simulink model "sdl_gear_efficiency"  (R2019b)
settings: Solver=VariableStepAuto  StartTime=0.0  StopTime=10  FixedStep=0.01  RelTol=1e-3  AbsTol=1e-3  EnableMultiTasking=on
undefined symbols (not defined in the file): sigbuilder_block
libraries: fl_lib x6, nesl_utility x5, sdl_lib x3
CloseFcn:
  | try,close(h1_sdl_gear_efficiency),end
  | clear h1_sdl_gear_efficiency
  | 
  | 
  | clear simlog_sdl_gear_efficiency
  | clear logsout_sdl_gear_efficiency
Description:
  | Gearbox Efficiency Measurement
settings Model: Creator=MathWorks  LastModifiedBy=JPark
settings SolverCC: AutoScaleAbsTol=off  MaxConsecutiveMinStep=5
settings DataIOCC: LimitDataPoints=on  MaxDataPoints=10000  SaveOutput=off  DSMLogging=off  SaveTime=off  ReturnWorkspaceOutputs=off  SignalLoggingName=logsout_sdl_gear_efficiency
settings OptimizationCC: ExpressionDepthLimit=2147483647  EfficientMapNaN2IntZero=off  LifeSpan=inf
settings DebuggingCC: StateNameClashWarn=warning  PregeneratedLibrarySubsystemCodeDiagnostic=none  SFUnexpectedBacktrackingDiag=warning  SFNoUnconditionalDefaultTransitionDiag=warning  SFExecutionAtInitializationDiag=none  ArithmeticOperatorsInVariantConditions=warning
settings HardwareCC: ProdBitPerPointer=32  ProdBitPerSizeT=32  ProdBitPerPtrDiffT=32  ProdLargestAtomicFloat=None  ProdIntDivRoundTo=Undefined  ProdEndianess=Unspecified  ProdWordSize=32  ProdHWDeviceType=32-bit Generic
settings ModelReferenceCC: PropagateSignalLabelsOutOfModel=off
settings SFSimCC: SimUseLocalCustomCode=off  CustomCodeUndefinedFunction=UseInterfaceOnly
settings RTWCC: RTWUseLocalCustomCode=off
settings CodeAppCC: StateflowObjectComments=on
settings GRTTargetCC: TargetLangStandard=C89/C90 (ANSI)  GeneratePreprocessorConditionals=Disable all  CombineOutputUpdateFcns=off  GRTInterface=on
settings ConfigComp: CovMetricSettings=dw  CovHtmlReporting=on  CovSaveCumulativeToWorkspaceVar=on  CovSaveSingleToWorkspaceVar=on  CovShowResultsExplorer=off  CovExternalEMLEnable=off
settings SimscapeCC: SimscapeLogType=all  SimscapeLogSimulationStatistics=on  SimscapeLogName=simlog_sdl_gear_efficiency  SimscapeLogDataHistory=10000

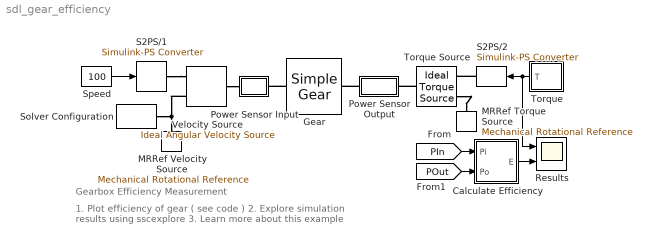
== system sdl_gear_efficiency ==
  note: Gearbox Efficiency Measurement
  note: 1. Plot efficiency of gear ( see code )
      | 2. Explore simulation results using sscexplore
      | 3. Learn more about this example
  Calculate Efficiency : Subsystem
  Gear : sdl_lib/Gears/Simple Gear  ratio=6.3  rotation_direction=1  friction_model=3  T_noload=2.4 N*m  T_nom=150 N*m  efficiency_nom=0.8  efficiency=0.8  mu_visc=[ 1e-5 1e-5 ] N*m/(rad/s)  w_thr=0.01 rad/s  pwr_thr=0.001 W  enable_faults=simscape.enum.onoff.off  efficiency_fault=0.05  external_fault=simscape.enum.onoff.off  temporal_fault=simscape.enum.onoff.off  fault_time=5 s  fault_angles=pi / 12 rad  report_fault=1  temperature_TLU=[ 280 300 320 ] K  load_TLU=[ 1 5 10 ] N*m  efficiency_TLU=[ 0.95 0.9 0.85 ]  efficiency_TLU2=[ 0.85 0.8 0.75; 0.95 0.9 0.85; 0.85 0.8 0.7 ]  thermal_mass=50 J/K  T_init=300 K
      settings: SourceProductName=Simscape Driveline
      settings: AttributesFormatString=|
      | Nominal Efficiency: %<efficiency_nom>
      | Nominal Output Torque: %<T_nom> %<T_nom_unit>
  MRRef Torque Source : fl_lib/Mechanical/Rotational Elements/Mechanical Rotational Reference
  MRRef Velocity Source : fl_lib/Mechanical/Rotational Elements/Mechanical Rotational Reference
  Power Sensor Input : Subsystem
      mask Display: disp('PIn');
  Power Sensor Output : Subsystem
      mask Display: disp('POut');
  Results : Scope  NumInputPorts=2
  S2PS/1 : nesl_utility/Simulink-PS Converter  PhysicalDomain=network_engine_domain  SubClassName=ps_input  LeftPortType=input  RightPortType=output  PseudoPeriodic=off  Frequencies=[]  NoiseDistribution=none  NoiseParameters=[]  Unit=rad/s  AffineConversion=off  FilteringAndDerivatives=zero  SimscapeFilterOrder=1  InputFilterTimeConstant=.001  UdotUserProvided=0
  S2PS/2 : nesl_utility/Simulink-PS Converter  PhysicalDomain=network_engine_domain  SubClassName=ps_input  LeftPortType=input  RightPortType=output  PseudoPeriodic=off  Frequencies=[]  NoiseDistribution=none  NoiseParameters=[]  Unit=N*m  AffineConversion=off  FilteringAndDerivatives=zero  SimscapeFilterOrder=1  InputFilterTimeConstant=.001  UdotUserProvided=0
  Solver Configuration : nesl_utility/Solver Configuration  PhysicalDomain=network_engine_domain  SubClassName=solver  LeftPortType=input  RightPortType=generic  Tones=[]  Harmonics=[]  SimulateNoise=off  Profile=off  UseLocalSampling=off  EnableSwitchedLinearOptims=on  FrequencyDomain=off  UseCCode=off  RelTol=0.001  AbsTol=1e-06  MinStep=1e-09  ToWorkspace=off  RevertToSquareIcSolve=off  NumHomotopyIterations=100  PhasorMode=off  PhasorModeNumHarmonics=1  DoDC=off  ResidualTolerance=1e-9  UseLocalSolver=off  LocalSolverChoice=NE_PARTITIONING_ADVANCER  LocalSolverSampleTime=0.01  DoFixedCost=off  MaxNonlinIter=3  MaxModeIter=2  LinearAlgebra=auto  EquationFormulation=NE_TIME_EF  DelaysMemoryBudget=1024  AutomaticFiltering=on  FilteringTimeConstant=0.001  PartitionStorageMethod=EXHAUSTIVE  PartitionMemoryBudget=1024  PartitionMethod=ROBUST
  Speed : Constant  Value=100
  Torque : Subsystem  Tag=STV Subsys  LoadFcn=sigbuilder_block('load');  StartFcn=sigbuilder_block('start');  StopFcn=sigbuilder_block('stop');  ClipboardFcn=sigbuilder_block('clipboard');  mask(Sigbuilder block){tuvar=[0:10]}
      mask help: Sigbuilder GUI
      mask init:
      | if ~strcmp(get_param(bdroot(gcbh),'SimulationStatus'),'stopped') tuvar = sigbuilder_block('maskInit'); end
      settings: CopyFcn=sigbuilder_block('copy');  DeleteFcn=sigbuilder_block('delete');  ModelCloseFcn=sigbuilder_block('modelClose');  PreSaveFcn=sigbuilder_block('preSave');  PauseFcn=sigbuilder_block('pause')  ContinueFcn=sigbuilder_block('continue')  NameChangeFcn=sigbuilder_block('namechange');  OpenFcn=sigbuilder_block('open',[301.2 157.5 550.2 398.4 ]);  CloseFcn=sigbuilder_block('close');
      mask Display: plot(0, 0, 100, 100,[2, 2, 32, 32, 2], [68, 8, 8, 68, 68],[32, 2], [38, 38], [32, 19, 2],[53, 60, 44], [32, 17, 17, 2],[16, 16, 31, 31]);txt = getActiveGroup(gcbh);text(2, 100, txt,'verticalAlignment', 'top');
  Torque Source : fl_lib/Mechanical/Mechanical Sources/Ideal Torque Source
  Velocity Source : fl_lib/Mechanical/Mechanical Sources/Ideal Angular Velocity Source
  wires:
  Speed/1 -> S2PS/1/1
  [PIn] -> Calculate Efficiency/1(Pi)
  Torque/1(T) -> Results/1, S2PS/2/1
  [POut] -> Calculate Efficiency/2(Po)
  Calculate Efficiency/1(E) -> Results/2
  connections:
  Velocity Source/LConn1 -- Power Sensor Input/LConn1
  S2PS/1/RConn1 -- Velocity Source/RConn1
  Velocity Source/RConn2 -- Solver Configuration/RConn1 -- MRRef Velocity Source/LConn1
  Torque Source/RConn2 -- MRRef Torque Source/LConn1
  Gear/LConn1 -- Power Sensor Input/RConn1
  Power Sensor Output/LConn1 -- Gear/RConn1
  S2PS/2/RConn1 -- Torque Source/RConn1
  Torque Source/LConn1 -- Power Sensor Output/RConn1

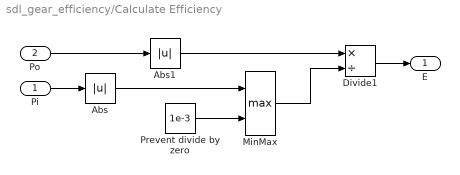
== system sdl_gear_efficiency/Calculate Efficiency ==
  Pi : Inport
  Po : Inport  Port=2
  Abs : Abs
  Abs1 : Abs
  Divide1 : Product  Inputs=*/
  MinMax : MinMax  Function=max  Inputs=2
  Prevent divide by zero : Constant  Value=1e-3
  E : Outport  VectorParamsAs1DForOutWhenUnconnected=off
  wires:
  Prevent divide by zero/1 -> MinMax/2
  MinMax/1 -> Divide1/2
  Abs/1 -> MinMax/1
  Abs1/1 -> Divide1/1
  Po/1 -> Abs1/1
  Pi/1 -> Abs/1
  Divide1/1 -> E/1

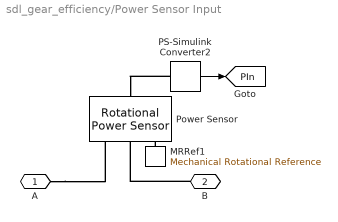
== system sdl_gear_efficiency/Power Sensor Input ==
  MRRef1 : fl_lib/Mechanical/Rotational Elements/Mechanical Rotational Reference
  PS-Simulink Converter2 : nesl_utility/PS-Simulink Converter  PhysicalDomain=network_engine_domain  SubClassName=ps_output  LeftPortType=input  RightPortType=output  PseudoPeriodic=off  Frequencies=[]  Unit=W  AffineConversion=off
  Power Sensor : sdl_lib/Sensors/Rotational Power Sensor  measurement_type=1  averaging_period=1 s  max_frequency=1000 Hz  max_speed=1000 rpm
      settings: SourceProductName=Simscape Driveline  SourceProductBaseCode=LD  InternalSimscapePortConfiguration="{\"Bottom\":[],\"Left\":[{\"id\":\"S\",\"label\":\"S\",\"type\":\"foundation.mechanical.rotational.rotational\"},{\"id\":\"R\",\"label\":\"R\",\"type\":\"foundation.mechanical.rotational.rotational\"},{\"id\":\"C\",\"label\":\"C\",\"type\":\"foundation.mechanical.rotational.rotational\"}],\"Right\":[{\"id\":\"P\",\"label\":\"P\",\"type\":\"output\"}],\"Top\":[]}"
  A : PMIOPort  Side=Left
  B : PMIOPort  Port=2  Side=Right
  tag scope: PIn=global
  wires:
  PS-Simulink Converter2/1 -> [PIn]
  connections:
  MRRef1/LConn1 -- Power Sensor/LConn3
  PS-Simulink Converter2/LConn1 -- Power Sensor/RConn1
  A/RConn1 -- Power Sensor/LConn1
  B/RConn1 -- Power Sensor/LConn2

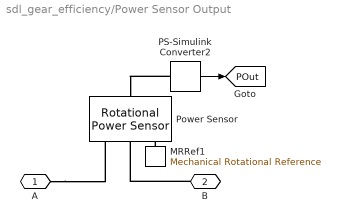
== system sdl_gear_efficiency/Power Sensor Output ==
  MRRef1 : fl_lib/Mechanical/Rotational Elements/Mechanical Rotational Reference
  PS-Simulink Converter2 : nesl_utility/PS-Simulink Converter  PhysicalDomain=network_engine_domain  SubClassName=ps_output  LeftPortType=input  RightPortType=output  PseudoPeriodic=off  Frequencies=[]  Unit=W  AffineConversion=off
  Power Sensor : sdl_lib/Sensors/Rotational Power Sensor  measurement_type=1  averaging_period=1 s  max_frequency=1000 Hz  max_speed=1000 rpm
      settings: SourceProductName=Simscape Driveline  SourceProductBaseCode=LD  InternalSimscapePortConfiguration="{\"Bottom\":[],\"Left\":[{\"id\":\"S\",\"label\":\"S\",\"type\":\"foundation.mechanical.rotational.rotational\"},{\"id\":\"R\",\"label\":\"R\",\"type\":\"foundation.mechanical.rotational.rotational\"},{\"id\":\"C\",\"label\":\"C\",\"type\":\"foundation.mechanical.rotational.rotational\"}],\"Right\":[{\"id\":\"P\",\"label\":\"P\",\"type\":\"output\"}],\"Top\":[]}"
  A : PMIOPort  Side=Left
  B : PMIOPort  Port=2  Side=Right
  tag scope: POut=global
  wires:
  PS-Simulink Converter2/1 -> [POut]
  connections:
  B/RConn1 -- Power Sensor/LConn2
  A/RConn1 -- Power Sensor/LConn1
  PS-Simulink Converter2/LConn1 -- Power Sensor/RConn1
  MRRef1/LConn1 -- Power Sensor/LConn3

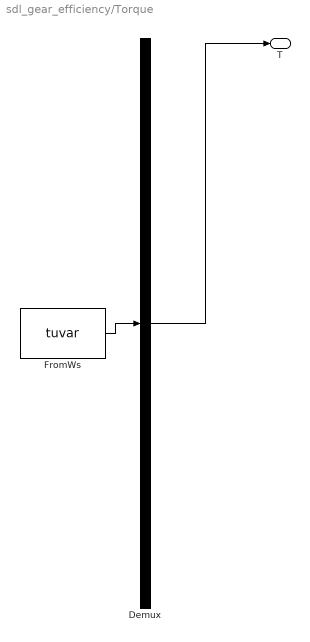
== system sdl_gear_efficiency/Torque ==
  Demux : Demux  Tag=STV Demux  Outputs=1
  FromWs : FromWorkspace  Tag=STV FromWs  VariableName=tuvar  SampleTime=0
      SigBuilderData=|
      | common.afterFinalStr = 'Extrapolate'
      | common.sampleTime = 0
      | dataSet.timeRange = [0 10]
      | dataSet.name = 'Group 1'
      | sbobj.Groups.Name = 'Group 1'
      | sbobj.Groups.Signals.Name = 'T'
      | sbobj.Groups.Signals.XData = [0 5 10]
      | sbobj.Groups.Signals.YData = [-0.001 -150 -0.001]
  T : Outport  Tag=STV Outport  VectorParamsAs1DForOutWhenUnconnected=off
  wires:
  Demux/1 -> T/1
  FromWs/1 -> Demux/1
